simulink model "untitled4"  (R2018b)
settings: Solver=VariableStepAuto  StartTime=0.0  StopTime=5  RelTol=1e-3
libraries: commfilt2 x2, commdigbbndpm3 x2, commrandsrc3 x1, commsink2 x1
settings Model: Creator=nhat  LastModifiedBy=nhat

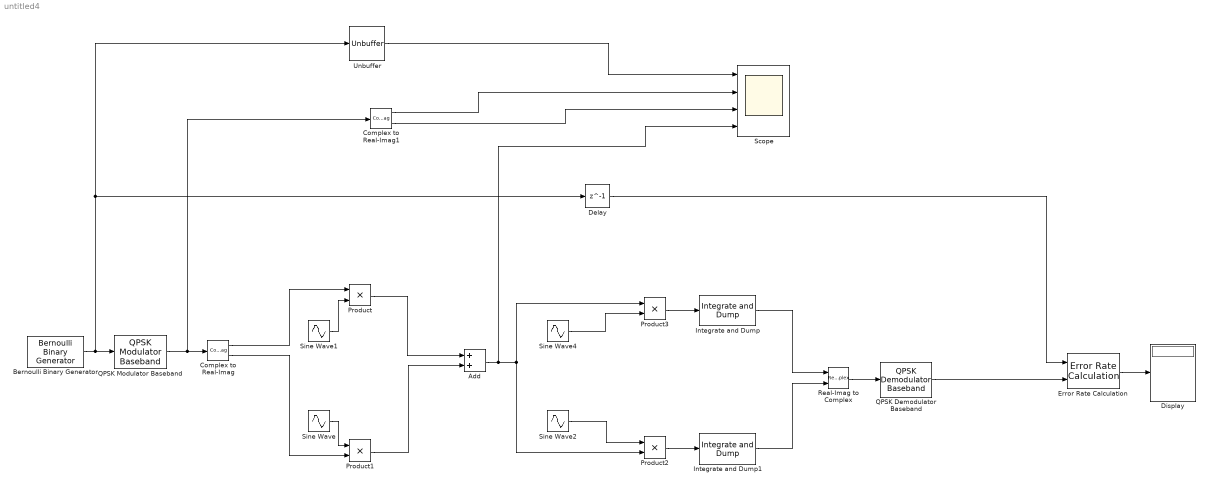
== system untitled4 ==
  Add : Sum
  Bernoulli Binary Generator : commrandsrc3/Bernoulli Binary Generator  ProbabilityOfZero=0.5  SeedSource=Auto  Seed=0  SampleTime=1/2000  SamplesPerFrame=2  OutputDataType=double  SimulateUsing=Interpreted execution
  Complex to Real-Imag : ComplexToRealImag
  Complex to Real-Imag1 : ComplexToRealImag
  Delay : Delay  DelayLength=1
  Display : Display
  Error Rate Calculation : commsink2/Error Rate Calculation  N=0  st_delay=0  cp_mode=Entire frame  subframe=[]  PMode=Port  WsName=ErrorVec  RsMode2=off  stop=off  numErr=100  maxBits=1e6
  Integrate and Dump : commfilt2/Integrate and Dump  obssamples=100  offsetsamples=0  nodump=off  roundingMode=Floor  overflowMode=off  outputDataTypeStr=Inherit: Same as accumulator  outputLastDataTypeStr=Inherit: Same as accumulator
      settings: SourceProductName=Communications System Toolbox
  Integrate and Dump1 : commfilt2/Integrate and Dump  obssamples=100  offsetsamples=0  nodump=off  roundingMode=Floor  overflowMode=off  outputDataTypeStr=Inherit: Same as accumulator  outputLastDataTypeStr=Inherit: Same as accumulator
      settings: SourceProductName=Communications System Toolbox
  Product{,1..3} (4 alike) : Product
  QPSK Demodulator Baseband : commdigbbndpm3/QPSK Demodulator Baseband  OutType=Bit  DecType=Hard decision  VarSource=Dialog  Variance=1  Dec=Gray  Ph=pi/4  outDtype1=Inherit via internal rule  outDtype2=Inherit via internal rule  derotateFactorWordLen=16  derotateFactorDataTypeStr=Inherit: Same word length as input  derotateFactorLastDataTypeStr=Inherit: Same word length as input
  QPSK Modulator Baseband : commdigbbndpm3/QPSK Modulator Baseband  InType=Bit  Enc=Gray  Ph=pi/4  outDtype=double  outWordLen=16  outUDDataType=sfix(16)  outFracLenMode=Best precision  outFracLen=15  outDataTypeStr=double  outLastDataTypeStr=double
  Real-Imag to Complex : RealImagToComplex
  Scope : Scope  NumInputPorts=4
  Sine Wave : Sin  Frequency=10000*2*pi  Phase=pi/2  SampleTime=1/100000
  Sine Wave1 : Sin  Frequency=10000*2*pi  SampleTime=1/100000
  Sine Wave2 : Sin  Frequency=10000*2*pi  Phase=pi/2  SampleTime=1/100000
  Sine Wave4 : Sin  Frequency=10000*2*pi  SampleTime=1/100000
  Unbuffer : Unbuffer
  wires:
  Bernoulli Binary Generator/1 -> Unbuffer/1, Delay/1, QPSK Modulator Baseband/1
  QPSK Modulator Baseband/1 -> Complex to Real-Imag1/1, Complex to Real-Imag/1
  Complex to Real-Imag/1 -> Product/1
  Complex to Real-Imag/2 -> Product1/2
  Sine Wave1/1 -> Product/2
  Sine Wave/1 -> Product1/1
  Product/1 -> Add/1
  Product1/1 -> Add/2
  Sine Wave2/1 -> Product2/1
  Sine Wave4/1 -> Product3/2
  Add/1 -> Scope/4, Product3/1, Product2/2
  Product3/1 -> Integrate and Dump/1
  Product2/1 -> Integrate and Dump1/1
  Integrate and Dump/1 -> Real-Imag to Complex/1
  Integrate and Dump1/1 -> Real-Imag to Complex/2
  Real-Imag to Complex/1 -> QPSK Demodulator Baseband/1
  QPSK Demodulator Baseband/1 -> Error Rate Calculation/2
  Error Rate Calculation/1 -> Display/1
  Delay/1 -> Error Rate Calculation/1
  Complex to Real-Imag1/2 -> Scope/3
  Complex to Real-Imag1/1 -> Scope/2
  Unbuffer/1 -> Scope/1
